simulink model "circuitbd"  (Simulink 7.4)
settings: Solver=ode45  StartTime=0.0  StopTime=10.0  RelTol=1e-3
values from neighbouring files (symbols this model uses):
  C = [1 0; 0 1; 1 -R; 0 R; 0 -1]    [ssmodels.m]
  L = 1    [ssmodels.m]
  R = 1    [ssmodels.m]
settings Model: Creator=eechris  LastModifiedBy=eechris

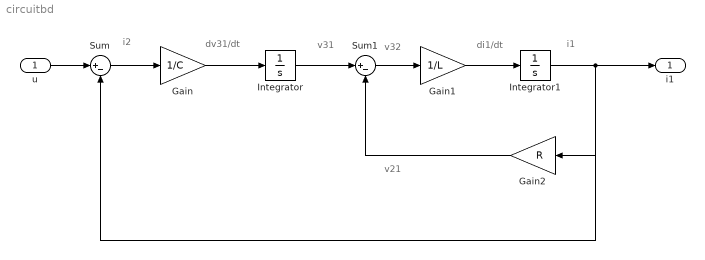
== system circuitbd ==
  note: i2
  note: dv31/dt
  note: v31
  note: v32
  note: di1/dt
  note: i1
  note: v21
  u : Inport  OutDataType=fixdt(1, 16)  OutScaling=2^0
  Gain : Gain  Gain=1/C  ParameterDataType=fixdt(1, 16)  ParameterScaling=2^0  OutDataType=fixdt(1, 16)  OutScaling=2^0
  Gain1 : Gain  Gain=1/L  ParameterDataType=fixdt(1, 16)  ParameterScaling=2^0  OutDataType=fixdt(1, 16)  OutScaling=2^0
  Gain2 : Gain  Gain=R  ParameterDataType=fixdt(1, 16)  ParameterScaling=2^0  OutDataType=fixdt(1, 16)  OutScaling=2^0
  Integrator : Integrator
  Integrator1 : Integrator
  Sum : Sum  Inputs=|+-  OutDataType=fixdt(1, 16)  OutScaling=2^0
  Sum1 : Sum  Inputs=|+-  OutDataType=fixdt(1, 16)  OutScaling=2^0
  i1 : Outport  OutDataType=fixdt(1, 16)  OutScaling=2^0
  wires:
  u/1 -> Sum/1
  Sum/1 -> Gain/1
  Gain/1 -> Integrator/1
  Integrator/1 -> Sum1/1
  Sum1/1 -> Gain1/1
  Gain1/1 -> Integrator1/1
  Gain2/1 -> Sum1/2
  Integrator1/1 -> i1/1, Gain2/1, Sum/2
